simulink model "m03"  (R2023b)
settings: Solver=VariableStepAuto  StartTime=0.0  StopTime=10.0  RelTol=1e-3
settings Model: Creator=asus  LastModifiedBy=asus

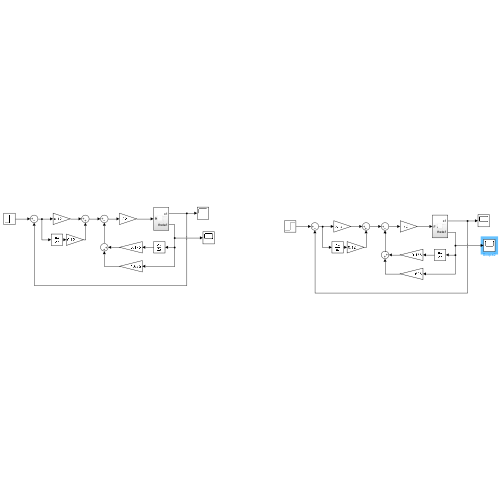
[thumbnail: Simulink's stored preview of the top-level diagram]
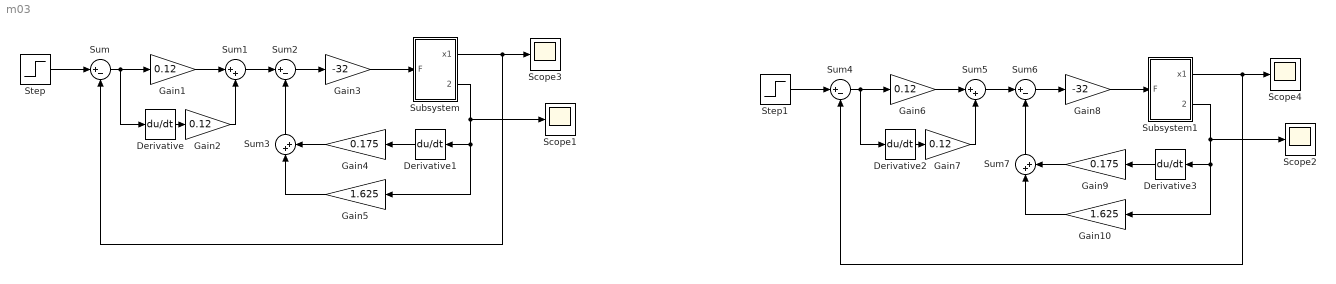
== system m03 ==
  Derivative{,1..3} (4 alike) : Derivative
  Gain{1..2,6..7} (4 alike) : Gain  Gain=0.12
  Gain10 : Gain  Gain=1.625
  Gain3 : Gain  Gain=-32
  Gain4 : Gain  Gain=0.175
  Gain5 : Gain  Gain=1.625
  Gain8 : Gain  Gain=-32
  Gain9 : Gain  Gain=0.175
  Scope{1..4} (4 alike) : Scope
  Step : Step  After=0.1  SampleTime=0
  Step1 : Step  After=0.1  SampleTime=0
  Subsystem : Subsystem
  Subsystem1 : Subsystem
  Sum{,2,4,6} (4 alike) : Sum  Inputs=|+-
  Sum{1,3,5,7} (4 alike) : Sum  Inputs=|++
  wires:
  Gain3/1 -> Subsystem/1(F)
  Derivative/1 -> Gain2/1
  Gain4/1 -> Sum3/2
  Sum/1 -> Derivative/1, Gain1/1
  Subsystem/1(x1) -> Scope3/1, Sum/2
  Step/1 -> Sum/1
  Gain2/1 -> Sum1/2
  Sum3/1 -> Sum2/2
  Derivative1/1 -> Gain4/1
  Subsystem/2(theta1) -> Scope1/1, Derivative1/1, Gain5/1
  Sum2/1 -> Gain3/1
  Sum1/1 -> Sum2/1
  Gain1/1 -> Sum1/1
  Gain5/1 -> Sum3/1
  Gain10/1 -> Sum7/1
  Gain6/1 -> Sum5/1
  Sum5/1 -> Sum6/1
  Sum6/1 -> Gain8/1
  Subsystem1/2(theta1) -> Gain10/1, Derivative3/1, Scope2/1
  Derivative3/1 -> Gain9/1
  Sum7/1 -> Sum6/2
  Gain7/1 -> Sum5/2
  Step1/1 -> Sum4/1
  Subsystem1/1(x1) -> Sum4/2, Scope4/1
  Sum4/1 -> Gain6/1, Derivative2/1
  Gain9/1 -> Sum7/2
  Derivative2/1 -> Gain7/1
  Gain8/1 -> Subsystem1/1(F)

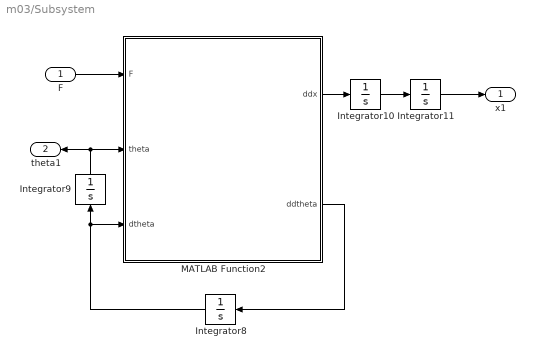
== system m03/Subsystem ==
  F : Inport
  Integrator{8..11} (4 alike) : Integrator
  MATLAB Function2 : MATLAB Function  TreatAsAtomicUnit=on
  x1 : Outport
  theta1 : Outport  Port=2
  wires:
  Integrator9/1 -> MATLAB Function2/2(theta), theta1/1
  Integrator8/1 -> MATLAB Function2/3(dtheta), Integrator9/1
  MATLAB Function2/1(ddx) -> Integrator10/1
  F/1 -> MATLAB Function2/1(F)
  Integrator10/1 -> Integrator11/1
  MATLAB Function2/2(ddtheta) -> Integrator8/1
  Integrator11/1 -> x1/1

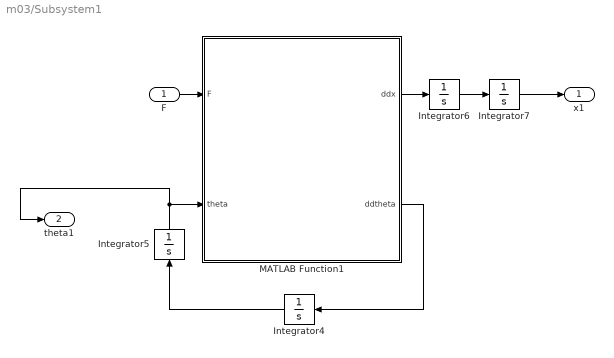
== system m03/Subsystem1 ==
  F : Inport
  Integrator{4..7} (4 alike) : Integrator
  MATLAB Function1 : MATLAB Function  TreatAsAtomicUnit=on
  x1 : Outport
  theta1 : Outport  Port=2
  wires:
  Integrator5/1 -> theta1/1, MATLAB Function1/2(theta)
  Integrator7/1 -> x1/1
  F/1 -> MATLAB Function1/1(F)
  MATLAB Function1/1(ddx) -> Integrator6/1
  Integrator4/1 -> Integrator5/1
  MATLAB Function1/2(ddtheta) -> Integrator4/1
  Integrator6/1 -> Integrator7/1

== matlab function m03/Subsystem1/MATLAB Function1 ==
  data: F input; ddx output; theta input; ddtheta output
function [ddx,ddtheta] = fcn(F,theta)

ddx = -6*theta + 0.8*F;
ddtheta = 40*theta-2.0*F;

== matlab function m03/Subsystem/MATLAB Function2 ==
  data: F input; ddx output; theta input; dtheta input; ddtheta output
function [ddx,ddtheta] = fcn(F,theta,dtheta)

ddx = 0.12*F + 0.036*sin(theta)*dtheta^2 - 0.9*sin(theta)*cos(theta);
ddx = ddx / ( 0.24 - 0.09*cos(theta)^2 );

ddtheta = 0.3*cos(theta)*F + 0.09*sin(theta)*cos(theta)*dtheta^2 - 6*sin(theta);
ddtheta = ddtheta / ( -0.24 + 0.09*cos(theta)^2 );
